simulink model "main"  (R2020b)
settings: Solver=ode23tb  StartTime=0.0  StopTime=20  FixedStep=0.0005  MaxStep=0.005  RelTol=1e-3  AbsTol=1e-3
StartFcn:
  | tic;
StopFcn:
  | Elapsed_Sim_Time = toc;
  | disp(['Elapsed Sim Time = ' num2str(Elapsed_Sim_Time)]);
model workspace (MATLAB code in the model file):
  | floor_l = 1.0900;
  | floor_d = 0.0100;
  | 
  | % PART
  | model_idx = 0;
  | model_dims = [0.06 0.06 0.06;
  |      0.02 0.05 0.07;
  |      0.04 0.04 0.10;
  |      0.05 0.05 0.05;
  |      0.10 0.08 0.08];
  | % distance between models on the conveyor belt
  | model_d = 0.12;
  | % distance to push models forwards in the -y dir (towards the box)
  | model_push = 0.2;
  | 
  | % BELT
  | belt_w = 0.1000;
  | belt_l = 1.2000;
  | belt_h = 0.0200;
  | belt_in_offset = [0 0.8000 0.0100];
  | 
  | container_belt_h = 0.02;
  | container_belt_l = 2.0;
  | container_belt_w = 0.2;
  | container_belt_offset = [-0.5050 0 -0.020];
  | 
  | belt_spd = 0.1;
  | 
  | % Model
  | cube_d = 0.06;
  | cube_z_off = belt_in_offset(3) + (container_belt_h / 2) + 0.001;
  | cube_z_offs = (model_dims(:,3) / 2) + cube_z_off;
  | 
  | % Container dimensions
  | % len, width, height are INTERNAL (Changed because most things were using internal anyway and it's 4am and we just need a working demo)
  | % Dimensions
  | container_len = 0.2;
  | container_width = 0.15;
  | container_height = 0.15;
  | container_thickness = 0.005;
  | 
  | 
  | % ????
  | cube_con_rsph = 0.003;
  | 
  | cube_con_k = 1000000;
  | cube_con_b = 1000;
  | 
  | finger_con_x = 0.01;
  | finger_con_y = 0.01;
  | finger_con_z = 5e-4;
  | finger_con_rsph = 5.0000e-04;
  | finger_con_muk = 0.05;
  | finger_con_mus = 0.07;
  | finger_con_vth = 1e-3;
  | 
  | finger_l = 0.4;
  | finger_w = 0.03;
  | finger_t = 0.01;
undefined symbols (not defined in the file): Bottom, Extr_Data_LinkHoles, Part1, Part2, Part3, Part4, Part5, point1, point2, point3, Side1, Side2, Side3, Side4, X, Y, Z
libraries: sm_lib x113, nesl_utility x35, Parts_Lib x10, Contact_Forces_Lib x6, sm_delta_robot_lib x1
(part 5 of 5)

== matlab function main/Image Processor/Optimiser Data ==
  data: model_positions input; model_id input; model_dims input; container_interior_bottom_left input; part_mesh output; container_mesh output; contents_mesh output; container_interior_top_right input
function [part_mesh, container_mesh, contents_mesh] = get_optimiser_data(model_positions, model_id, model_dims, container_interior_bottom_left, container_interior_top_right)

part_mesh_const = model_dims(model_id, 1:3) / 2;
model = model_positions((model_id*3-2): model_id*3);
part_mesh = [
    (model(1) - part_mesh_const(1)), (model(2) - part_mesh_const(2)), (model(3) - part_mesh_const(3));
    (model(1) + part_mesh_const(1)), (model(2) + part_mesh_const(2)), (model(3) + part_mesh_const(3));
];


container_mesh = [
    min(container_interior_bottom_left, container_interior_top_right).';
    max(container_interior_bottom_left, container_interior_top_right).';
];



contents_mesh = zeros(2, 3, 6);
%get positions of all contents of container
for id = 1:5
    model_mesh_offsets = model_dims(id, 1:3) / 2;
    model_position = model_positions((id*3-2): id*3);
    model_mesh_pos = [
        (model_position(1) - model_mesh_offsets(1)), (model_position(2) - model_mesh_offsets(2)), (model_position(3) - 2 * model_mesh_offsets(3));
        (model_position(1) + model_mesh_offsets(1)), (model_position(2) + model_mesh_offsets(2)), (model_position(3))
        ];
    contents_mesh(:, :, id) = model_mesh_pos;
end

== matlab function main/Vacuum/MATLAB Function ==
  data: suction input; suctions output; model_idx input
function suctions = fcn(suction, model_idx)

suctions = [0 0 0 0 0];
suctions(model_idx) = suction;

== matlab function main/Image Processor/Get Current Object Position ==
  data: model_positions input; model_position output; model_id input
function model_position = get_position(model_positions, model_id)

model_position = [
    model_positions(model_id * 3 - 2)
    model_positions(model_id * 3 - 1)
    model_positions(model_id * 3)
];

== matlab function main/Optimiser/Optimiser Wrapper ==
  settings: updateMethod=DISCRETE  sampleTime=0.1
  data: packed_item_count output; box_points output; item_points output; item_points_length output; item_indices output; tetromino_dimensions output; part_index input; part_mesh input; output_position output; container_mesh input; contents_mesh input; next_box output; items_packed_start_index_in input; items_packed_start_index_out output
function [packed_item_count, box_points, item_points, item_points_length, item_indices, tetromino_dimensions, output_position, next_box, items_packed_start_index_out] = wrapper(part_index, part_mesh, container_mesh, contents_mesh, items_packed_start_index_in)
    % Compress contents of box that have been packed into a single array
    index = 0;
    packed_item_count = (part_index - items_packed_start_index_in);
    item_indices = zeros(1, size(contents_mesh, 3));
    item_points = zeros(1, size(contents_mesh, 1) * size(contents_mesh, 2) * size(contents_mesh, 3));
    for i_item = items_packed_start_index_in:packed_item_count
        item_indices(i_item) = index;
        for i_point = 1:size(contents_mesh, 1)
            for i_dim = 1:3
                index = index + 1;
                item_points(index) = contents_mesh(i_point, i_dim, i_item);
            end
        end
    end
    % Custom calculate used cells to eliminate need for variable sized arrays
    item_points_length = size(contents_mesh, 1) * size(contents_mesh, 2) * packed_item_count; 
    
    % Find bottom left and top right of inside of box
    min_box = min(container_mesh(1, :), container_mesh(2, :));
    max_box = max(container_mesh(1, :), container_mesh(2, :));
    box_points = [min_box(1) min_box(2) min_box(3) max_box(1) max_box(2) max_box(3)];
    
    % Find the dimensions of the tetromino to pack
    tetromino_dimensions = abs(part_mesh(2, :) - part_mesh(1, :));
    
    % Invoke
    keep_box = false;
    output_position = [-1; -1; -1];
    keep_box = coder.ceval("process_optimiser_main", box_points, item_points, item_points_length, item_indices, packed_item_count, tetromino_dimensions, coder.wref(output_position));
    next_box = not(keep_box);
    
    % Check output_position is set to something
    if and(and(output_position(1) == -1, output_position(2) == -1), output_position(3) == -1)
        disp("Ceval is playing up again :(");
    end
    
    % Change location returned
    output_offset = [tetromino_dimensions(1) / 2; tetromino_dimensions(2) / 2; tetromino_dimensions(3)];
    output_position = output_position + output_offset;
    
    % Forget packed items if next box was requested
    items_packed_start_index_out = items_packed_start_index_in;
    if next_box
        items_packed_start_index_out = part_index;
    end
